simulink subsystem "s1EMSSC"  (R2023b)
settings: Solver=VariableStepAuto  StartTime=0.0  StopTime=10.0  RelTol=1e-3
settings Model: Creator=The MathWorks, Inc.  LastModifiedBy=The MathWorks, Inc.

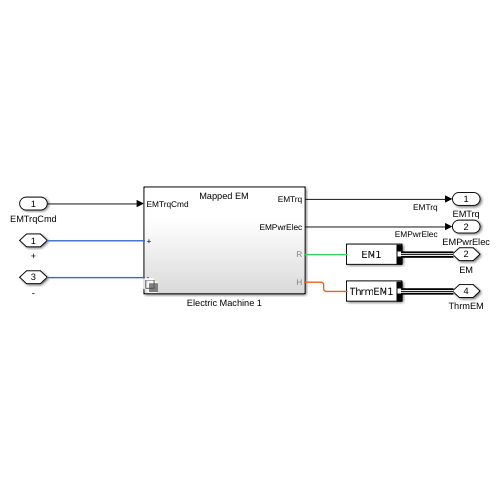
[thumbnail: Simulink's stored preview of the top-level diagram]
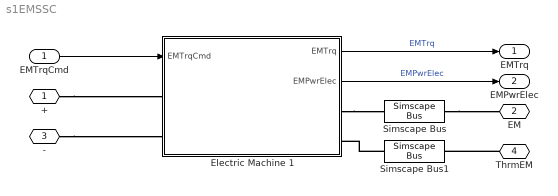
== system s1EMSSC ==
  EMTrqCmd : Inport
  Electric Machine 1 : Subsystem  Variant=on  VariantControlMode=label  LabelModeActiveChoice=Mapped EM
  Simscape Bus : SimscapeBus  HierarchyStrings=EM1
  Simscape Bus1 : SimscapeBus  HierarchyStrings=ThrmEM1
  + : PMIOPort  Side=Left
  EM : PMIOPort  Port=2  Side=Right
  - : PMIOPort  Port=3  Side=Left
  ThrmEM : PMIOPort  Port=4  Side=Right
  EMTrq : Outport
  EMPwrElec : Outport  Port=2
  wires:
  Electric Machine 1/1(EMTrq) -> EMTrq/1  "EMTrq"
  Electric Machine 1/2(EMPwrElec) -> EMPwrElec/1  "EMPwrElec"
  EMTrqCmd/1 -> Electric Machine 1/1(EMTrqCmd)
  connections:
  Simscape Bus1/LConn1 -- Electric Machine 1/RConn2
  ThrmEM/RConn1 -- Simscape Bus1/RConn1
  Electric Machine 1/RConn1 -- Simscape Bus/LConn1
  +/RConn1 -- Electric Machine 1/LConn1
  -/RConn1 -- Electric Machine 1/LConn2
  Simscape Bus/RConn1 -- EM/RConn1

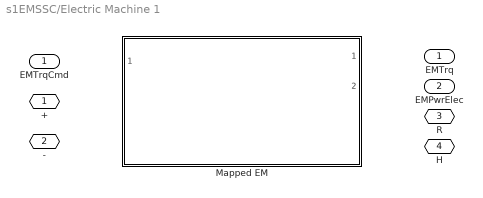
== system s1EMSSC/Electric Machine 1 ==
  EMTrqCmd : Inport
  Mapped EM : Subsystem  VariantControl=Mapped EM  ReferencedSubsystem=ElectricMachine1SSC
  + : PMIOPort  Side=Left
  - : PMIOPort  Port=2  Side=Left
  R : PMIOPort  Port=3  Side=Right
  H : PMIOPort  Port=4  Side=Right
  EMTrq : Outport  VectorParamsAs1DForOutWhenUnconnected=off
  EMPwrElec : Outport  Port=2  VectorParamsAs1DForOutWhenUnconnected=off
